simulink model "PID_GA_simulink"  (R2018a)
settings: Solver=FixedStepAuto  StartTime=0.0  StopTime=t_end  FixedStep=0.001  MinStep=1e-4  RelTol=1e-3
values from neighbouring files (symbols this model uses):
  Den = [1 12 24]    [GA_Ks.m]
  K = bestK    (= 0)    [GA_Ks.m]
  Kd = bestKd    (= 0)    [GA_Ks.m]
  Kp = bestKp    (= 0)    [GA_Ks.m]
  Num = [2]    [GA_Ks.m]
settings Model: SimulationMode=accelerator  Creator=Milosh Yokich  LastModifiedBy=Milosh Yokich

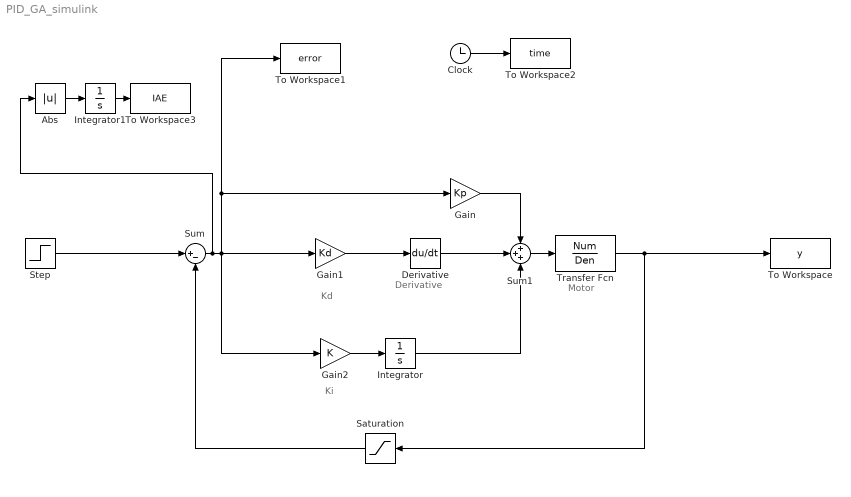
== system PID_GA_simulink ==
  note: Ki
  note: Derivative
  note: Motor
  note: Kd
  Abs : Abs
  Clock : Clock
  Derivative : Derivative  CoefficientInTFapproximation=0.001
  Gain : Gain  Gain=Kp
  Gain1 : Gain  Gain=Kd
  Gain2 : Gain  Gain=K
  Integrator : Integrator  AbsoluteTolerance=1e-4
  Integrator1 : Integrator
  Saturation : Saturate  UpperLimit=10  LowerLimit=-10
  Step : Step  Time=0  SampleTime=0
  Sum : Sum  Inputs=|+-
  Sum1 : Sum  Inputs=+++
  To Workspace : ToWorkspace  VariableName=y  SampleTime=-1
  To Workspace1 : ToWorkspace  VariableName=error  SampleTime=-1
  To Workspace2 : ToWorkspace  VariableName=time  SampleTime=-1
  To Workspace3 : ToWorkspace  VariableName=IAE  SampleTime=-1
  Transfer Fcn : TransferFcn  Numerator=Num  Denominator=Den
  wires:
  Step/1 -> Sum/1
  Gain1/1 -> Derivative/1
  Derivative/1 -> Sum1/2
  Clock/1 -> To Workspace2/1
  Transfer Fcn/1 -> To Workspace/1, Saturation/1
  Gain2/1 -> Integrator/1
  Integrator/1 -> Sum1/3
  Sum1/1 -> Transfer Fcn/1
  Sum/1 -> Abs/1, Gain2/1, Gain1/1, Gain/1, To Workspace1/1
  Abs/1 -> Integrator1/1
  Saturation/1 -> Sum/2
  Integrator1/1 -> To Workspace3/1
  Gain/1 -> Sum1/1
